simulink model "project2"  (R2022a)
settings: Solver=VariableStepAuto  StartTime=0.0  StopTime=2  RelTol=1e-3
libraries: spsSeriesRLCBranchLib x3, spsCurrentMeasurementLib x1, spsDiodeLib x1, spsDCVoltageSourceLib x1, spsMosfetLib x1, eePwmGenerator x1, spsVoltageMeasurementLib x1, spspowerguiLib x1
settings Model: Creator=Slava  LastModifiedBy=Slava
settings SolverCC: ZeroCrossAlgorithm=Adaptive
settings DebuggingCC: IgnoredZcDiagnostic=none

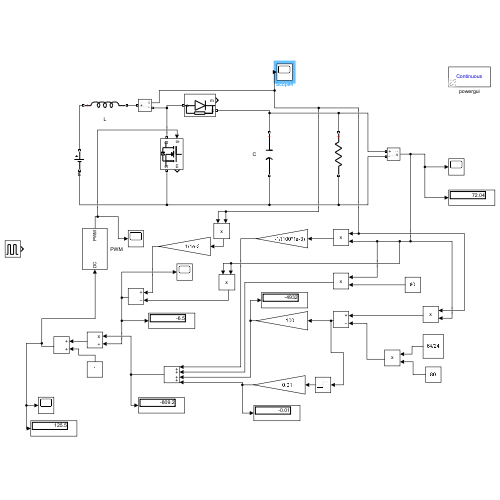
[thumbnail: Simulink's stored preview of the top-level diagram]
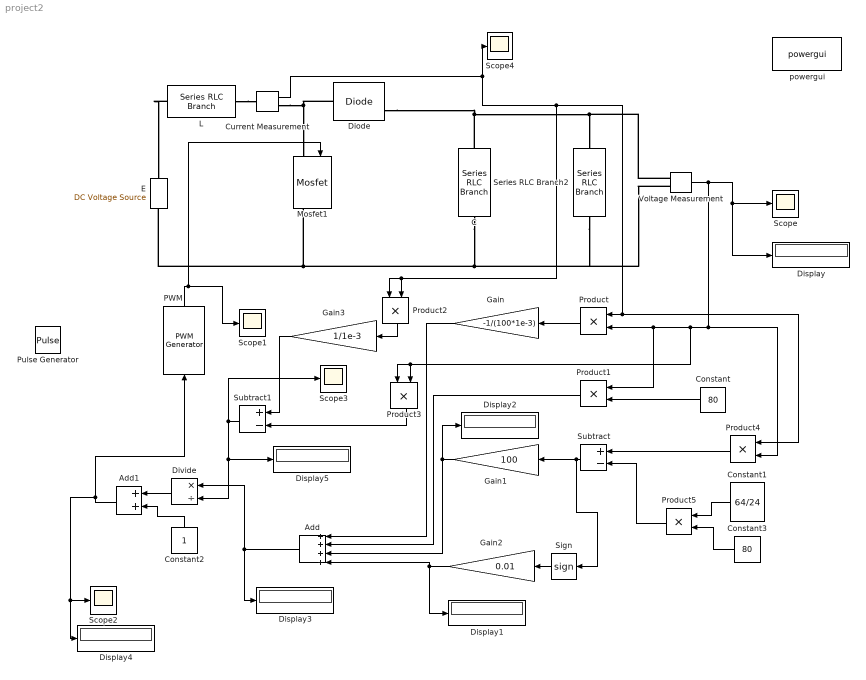
== system project2 ==
  Add : Sum  Inputs=++++
  Add1 : Sum
  C : spsSeriesRLCBranchLib/Series RLC Branch  LConnTagsString=__new0  RConnTagsString=__new0  BranchType=C  Resistance=1  Inductance=1e-3  SetiL0=off  InitialCurrent=0  Capacitance=1e-3  Setx0=off  InitialVoltage=0  Measurements=None
  Constant : Constant  Value=80
  Constant1 : Constant  Value=64/24
  Constant2 : Constant
  Constant3 : Constant  Value=80
  Current Measurement : spsCurrentMeasurementLib/Current Measurement  PhasorSimulation=off  OutputType=Complex  PSBequivalent=0
  Diode : spsDiodeLib/Diode  Ron=0.001  Lon=0  Vf=0.8  IC=0  UseSnubber=0  Rs=500  Cs=250e-9  Measurements=on
  Display{,1..5} (6 alike) : Display
  Divide : Product  Inputs=*/
  E : spsDCVoltageSourceLib/DC Voltage Source  Amplitude=24  Measurements=None
  Gain : Gain  Gain=-1/(100*1e-3)
  Gain1 : Gain  Gain=100
  Gain2 : Gain  Gain=0.01
  Gain3 : Gain  Gain=1/1e-3
  L : spsSeriesRLCBranchLib/Series RLC Branch  LConnTagsString=__new0  RConnTagsString=__new0  BranchType=L  Resistance=1  Inductance=1  SetiL0=off  InitialCurrent=0  Capacitance=1e-6  Setx0=off  InitialVoltage=0  Measurements=None
  Mosfet1 : spsMosfetLib/Mosfet  Ron=0.0001  Lon=0  Rd=0.0001  Vfd=0  IC=0  Rs=1e5  Cs=inf  Measurements=on
  "PWM " : eePwmGenerator/PWM Generator  CarrCount=Up  Tper=1/100  Tdelay=0  Ts=5e-5
  Product{,1..5} (6 alike) : Product
  Pulse Generator : DiscretePulseGenerator  PulseType=Time based  Period=1/100  PulseWidth=70
  Scope{,1..4} (5 alike) : Scope
  Series RLC Branch2 : spsSeriesRLCBranchLib/Series RLC Branch  LConnTagsString=__new0  RConnTagsString=__new0  BranchType=R  Resistance=100  Inductance=1e-3  SetiL0=off  InitialCurrent=0  Capacitance=1e-6  Setx0=off  InitialVoltage=0  Measurements=None
  Sign : Signum
  Subtract : Sum  Inputs=+-
  Subtract1 : Sum  Inputs=+-
  Voltage Measurement : spsVoltageMeasurementLib/Voltage Measurement  PhasorSimulation=off  OutputType=Complex  PSBequivalent=0
  powergui : spspowerguiLib/powergui  Priority=1  SimulationMode=Continuous  SampleTime=50e-6  frequency=60  Iterations=50  frequencyindice=0  Pbase=100e6  ErrMax=1e-4  UnitsV=kV  UnitsW=MW  buscounter=0  FunctionMessages=off  echomessages=off  EnableUseOfTLC=off  CurrentSourceSwitches=off  DisableSnubberDevices=off  DisableRonSwitches=off  DisableVfSwitches=off  DisplayEquations=off  AutomaticDiscreteSolvers=off  SolverType=Tustin/Backward Euler (TBE)  Interpol=off  ExternalGateDelay=off  methode=off  Ts=100  x0status=blocks  SPID=on  SwTol=0  HookPort=off  NonlinearTolerance=1e-4  nMaxIteration=100  ContinueOnMaxIteration=off  RestoreLinks=warning  ResistiveCurrentMeasurement=off  Frange=[0:2:500]  Ylog=off  Xlog=on  ShowGrid=off  save=off  variable=ZData  structure=0  ZoomFFT=off  StartTime=0.0  cycles=1  DisplayStyle=1  fundamental=60  FreqAxis=off  MaxFrequency=1000  frequencyindicesteady=1  RmsSteady=1  display=off
  wires:
  Voltage Measurement/1 -> Product3/2, Product3/1, Product1/1, Product/2, Product4/2, Display/1, Scope/1
  Current Measurement/1 -> Product2/1, Product2/2, Product4/1, Product/1, Scope4/1
  Product/1 -> Gain/1
  Constant/1 -> Product1/2
  Subtract/1 -> Sign/1, Gain1/1
  Sign/1 -> Gain2/1
  Product1/1 -> Add/2
  Gain1/1 -> Display2/1, Add/3
  Gain2/1 -> Display1/1, Add/4
  Gain/1 -> Add/1
  Product2/1 -> Gain3/1
  Gain3/1 -> Subtract1/1
  Product3/1 -> Subtract1/2
  Subtract1/1 -> Display5/1, Divide/2, Scope3/1
  Add/1 -> Display3/1, Divide/1
  Constant2/1 -> Add1/2
  Divide/1 -> Add1/1
  Add1/1 -> Display4/1, Scope2/1, "PWM "/1
  "PWM "/1 -> Mosfet1/1, Scope1/1
  Product4/1 -> Subtract/1
  Constant1/1 -> Product5/1
  Constant3/1 -> Product5/2
  Product5/1 -> Subtract/2
  connections:
  Diode/LConn1 -- Mosfet1/LConn1 -- Current Measurement/RConn1
  L/LConn1 -- E/RConn1
  C/RConn1 -- Series RLC Branch2/RConn1 -- Voltage Measurement/LConn2 -- E/LConn1 -- Mosfet1/RConn1
  C/LConn1 -- Diode/RConn1 -- Series RLC Branch2/LConn1 -- Voltage Measurement/LConn1
  L/RConn1 -- Current Measurement/LConn1
